simulink model "fixedPoint_model_q3"  (R2020b)
settings: Solver=FixedStepDiscrete  StartTime=0.0  StopTime=10  FixedStep=1/44100  RelTol=1e-3
settings Model: Creator=Faridodin  LastModifiedBy=Faridodin

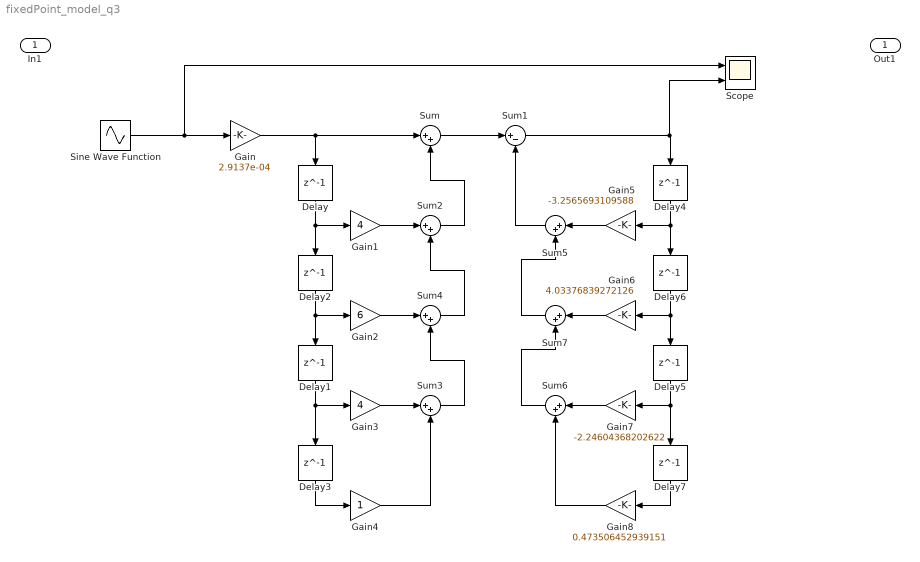
== system fixedPoint_model_q3 ==
  In1 : Inport
  Delay{,1..7} (8 alike) : Delay  DelayLength=1  InitialCondition=0
  Gain : Gain  Gain=2.9137e-04
  Gain1 : Gain  Gain=4
  Gain2 : Gain  Gain=6
  Gain3 : Gain  Gain=4
  Gain4 : Gain
  Gain5 : Gain  Gain=-3.2565693109588
  Gain6 : Gain  Gain=4.03376839272126
  Gain7 : Gain  Gain=-2.24604368202622
  Gain8 : Gain  Gain=0.473506452939151
  Scope : Scope  NumInputPorts=2
  Sine Wave Function : Sin  SampleTime=0
  Sum{,2..7} (7 alike) : Sum  Inputs=|++
  Sum1 : Sum  Inputs=|+-
  Out1 : Outport
  wires:
  Gain/1 -> Sum/1, Delay/1
  Sum/1 -> Sum1/1
  Delay/1 -> Delay2/1, Gain1/1
  Sum2/1 -> Sum/2
  Gain1/1 -> Sum2/1
  Gain2/1 -> Sum4/1
  Delay2/1 -> Delay1/1, Gain2/1
  Sum4/1 -> Sum2/2
  Delay1/1 -> Delay3/1, Gain3/1
  Gain3/1 -> Sum3/1
  Sum3/1 -> Sum4/2
  Delay3/1 -> Gain4/1
  Gain4/1 -> Sum3/2
  Gain8/1 -> Sum6/2
  Gain6/1 -> Sum7/1
  Delay6/1 -> Delay5/1, Gain6/1
  Sum6/1 -> Sum7/2
  Gain7/1 -> Sum6/1
  Gain5/1 -> Sum5/1
  Delay7/1 -> Gain8/1
  Delay5/1 -> Delay7/1, Gain7/1
  Sum7/1 -> Sum5/2
  Delay4/1 -> Delay6/1, Gain5/1
  Sum5/1 -> Sum1/2
  Sum1/1 -> Scope/2, Delay4/1
  Sine Wave Function/1 -> Scope/1, Gain/1
